simulink model "Regelungsmodell_Roboterarm"  (R2018b)
settings: Solver=VariableStepAuto  StartTime=0.0  StopTime=2  RelTol=1e-3
values from neighbouring files (symbols this model uses):
  konvert_i_torque = 0.11    [Aufgabe_3_Regler.m]
libraries: simulink x2, cstblocks x2
settings Model: Creator=jens  LastModifiedBy=jens

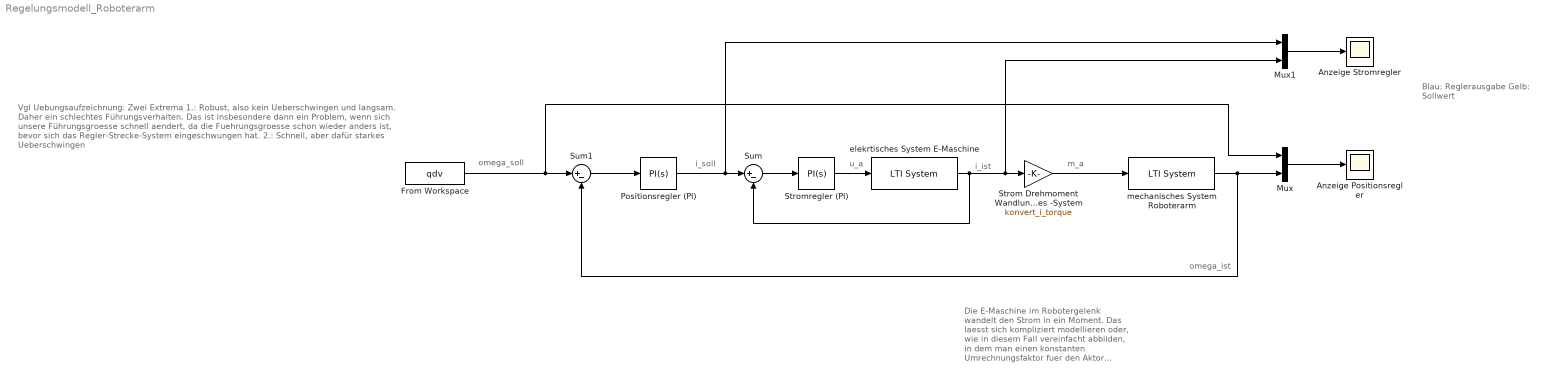
== system Regelungsmodell_Roboterarm ==
  note: Vgl Uebungsaufzeichnung:
      |
      | Zwei Extrema
      |
      | 1.: Robust, also kein Ueberschwingen und langsam. Daher ein schlechtes Führungsverhalten. Das ist insbesondere dann ein Problem, wenn sich unsere Führungsgroesse schnell aendert, da die Fuehrungsgroesse schon wieder anders ist, bevor sich das Regler-Strecke-System eingeschwungen hat.
      |
      | 2.: Schnell, aber dafür starkes Ueberschwingen
  note: m_a
  note: i_ist
  note: u_a
  note: i_soll
  note: omega_soll
  note: omega_ist
  note: Blau:
      | Reglerausgabe
      |
      | Gelb:
      | Sollwert
  note: Die E-Maschine im Robotergelenk wandelt den Strom in ein Moment. Das laesst sich kompliziert modellieren oder, wie in diesem Fall vereinfacht abbilden, in dem man einen konstanten Umrechnungsfaktor fuer den Aktor verwendet.
      | Das ist quasi die Schnittstelle zwischen dem elektrischen Modell und dem mechanischen Modell! Das gestellte Moment m_a ist ueber den Faktor 'konvert_i_torque' direkt proportional zum durch den Stromregler umgesetzten Strom
  Anzeige Positionsregler : Scope
  Anzeige Stromregler : Scope
  From Workspace : FromWorkspace  VariableName=qdv  SampleTime=0
  Mux : Mux  Inputs=2
  Mux1 : Mux  Inputs=2
  Positionsregler (PI) : simulink/Continuous/PID Controller  Controller=PI  Form=Parallel  TimeDomain=Continuous-time  SampleTime=-1  IntegratorMethod=Forward Euler  FilterMethod=Forward Euler  ControllerParametersSource=internal  P=0.150480850040603  I=3  D=0  UseFilter=on  N=100  TunerSelectOption=Transfer Function Based (PID Tuner App)  InitialConditionSource=internal  InitialConditionForIntegrator=0  InitialConditionForFilter=0  DifferentiatorICPrevScaledInput=0  ExternalReset=none  TrackingMode=off  Kt=1  LimitOutput=off  UpperSaturationLimit=inf  LowerSaturationLimit=-inf  LinearizeAsGain=on  AntiWindupMode=none  Kb=1  POutMin=[]  POutMax=[]  IOutMin=[]  IOutMax=[]  DOutMin=[]  DOutMax=[]  NOutMin=[]  NOutMax=[]  SumOutMin=[]  SumOutMax=[]  SaturationOutMin=[]  SaturationOutMax=[]  PParamMin=[]  PParamMax=[]  IParamMin=[]  IParamMax=[]  DParamMin=[]  DParamMax=[]  NParamMin=[]  NParamMax=[]  KbParamMin=[]  KbParamMax=[]  KtParamMin=[]  KtParamMax=[]  KbOutMin=[]  KbOutMax=[]  KtOutMin=[]  KtOutMax=[]  IntegratorOutMin=[]  IntegratorOutMax=[]  FilterOutMin=[]  FilterOutMax=[]  SumI1OutMin=[]  SumI1OutMax=[]  SumI2OutMin=[]  SumI2OutMax=[]  SumI3OutMin=[]  SumI3OutMax=[]  SumI4OutMin=[]  SumI4OutMax=[]  SumDOutMin=[]  SumDOutMax=[]  DifferentiatorOutMin=[]  DifferentiatorOutMax=[]  FilterDiffOutCoefMin=[]  FilterDiffOutCoefMax=[]  ReciprocalOutMin=[]  ReciprocalOutMax=[]  SumDenOutMin=[]  SumDenOutMax=[]  SumNumOutMin=[]  SumNumOutMax=[]  DivideOutMin=[]  DivideOutMax=[]  IntegratorContinuousStateAttributes=''  IntegratorStateMustResolveToSignalObject=off  IntegratorRTWStateStorageClass=Auto  FilterContinuousStateAttributes=''  FilterStateMustResolveToSignalObject=off  FilterRTWStateStorageClass=Auto  ParallelPVariant=InternalParameters  IdealPVariant=Disabled  IVariant=InternalParameters  DVariant=Disabled  IntegratorVariant=Continuous  SatVariant=Disabled  AWVariant=Passthrough  PCopyVariant=Disabled  TRVariant=Disabled  FdbkBlocksVariant=Forward  IdealPFdbkVariant=Disabled  SatFdbkVariant=Disabled  DerivativeFilterVariant=Disabled  NVariant=Disabled  NCopyVariant=Disabled_SignalSpec  FilterICVariant=Disabled  IntegratorICVariant=InternalICs  ExternalResetVariant=Disabled  TRSumVariant=Passthrough  SumFdbkVariant=Disabled  SumVariant=Sum_PI
  "Strom Drehmoment Wandlung - Schnittstelle elektrisches- und mechanisches -System " : Gain  Gain=konvert_i_torque
  Stromregler (PI) : simulink/Continuous/PID Controller  Controller=PI  Form=Parallel  TimeDomain=Continuous-time  SampleTime=-1  IntegratorMethod=Forward Euler  FilterMethod=Forward Euler  ControllerParametersSource=internal  P=0.3  I=3.5  D=0  UseFilter=on  N=100  TunerSelectOption=Transfer Function Based (PID Tuner App)  InitialConditionSource=internal  InitialConditionForIntegrator=0  InitialConditionForFilter=0  DifferentiatorICPrevScaledInput=0  ExternalReset=none  TrackingMode=off  Kt=1  LimitOutput=off  UpperSaturationLimit=inf  LowerSaturationLimit=-inf  LinearizeAsGain=on  AntiWindupMode=none  Kb=1  POutMin=[]  POutMax=[]  IOutMin=[]  IOutMax=[]  DOutMin=[]  DOutMax=[]  NOutMin=[]  NOutMax=[]  SumOutMin=[]  SumOutMax=[]  SaturationOutMin=[]  SaturationOutMax=[]  PParamMin=[]  PParamMax=[]  IParamMin=[]  IParamMax=[]  DParamMin=[]  DParamMax=[]  NParamMin=[]  NParamMax=[]  KbParamMin=[]  KbParamMax=[]  KtParamMin=[]  KtParamMax=[]  KbOutMin=[]  KbOutMax=[]  KtOutMin=[]  KtOutMax=[]  IntegratorOutMin=[]  IntegratorOutMax=[]  FilterOutMin=[]  FilterOutMax=[]  SumI1OutMin=[]  SumI1OutMax=[]  SumI2OutMin=[]  SumI2OutMax=[]  SumI3OutMin=[]  SumI3OutMax=[]  SumI4OutMin=[]  SumI4OutMax=[]  SumDOutMin=[]  SumDOutMax=[]  DifferentiatorOutMin=[]  DifferentiatorOutMax=[]  FilterDiffOutCoefMin=[]  FilterDiffOutCoefMax=[]  ReciprocalOutMin=[]  ReciprocalOutMax=[]  SumDenOutMin=[]  SumDenOutMax=[]  SumNumOutMin=[]  SumNumOutMax=[]  DivideOutMin=[]  DivideOutMax=[]  IntegratorContinuousStateAttributes=''  IntegratorStateMustResolveToSignalObject=off  IntegratorRTWStateStorageClass=Auto  FilterContinuousStateAttributes=''  FilterStateMustResolveToSignalObject=off  FilterRTWStateStorageClass=Auto  ParallelPVariant=InternalParameters  IdealPVariant=Disabled  IVariant=InternalParameters  DVariant=Disabled  IntegratorVariant=Continuous  SatVariant=Disabled  AWVariant=Passthrough  PCopyVariant=Disabled  TRVariant=Disabled  FdbkBlocksVariant=Forward  IdealPFdbkVariant=Disabled  SatFdbkVariant=Disabled  DerivativeFilterVariant=Disabled  NVariant=Disabled  NCopyVariant=Disabled_SignalSpec  FilterICVariant=Disabled  IntegratorICVariant=InternalICs  ExternalResetVariant=Disabled  TRSumVariant=Passthrough  SumFdbkVariant=Disabled  SumVariant=Sum_PI
  Sum : Sum  Inputs=|+-
  Sum1 : Sum  Inputs=|+-
  elekrtisches System E-Maschine : cstblocks/LTI System  sys=tf_motor  IC=[]
  mechanisches System Roboterarm : cstblocks/LTI System  sys=tf_arm  IC=[]
  wires:
  Sum/1 -> Stromregler (PI)/1
  Stromregler (PI)/1 -> elekrtisches System E-Maschine/1
  Positionsregler (PI)/1 -> Mux1/1, Sum/1
  From Workspace/1 -> Mux/1, Sum1/1
  Sum1/1 -> Positionsregler (PI)/1
  mechanisches System Roboterarm/1 -> Sum1/2, Mux/2
  Mux/1 -> Anzeige Positionsregler/1
  "Strom Drehmoment Wandlung - Schnittstelle elektrisches- und mechanisches -System "/1 -> mechanisches System Roboterarm/1
  Mux1/1 -> Anzeige Stromregler/1
  elekrtisches System E-Maschine/1 -> Mux1/2, "Strom Drehmoment Wandlung - Schnittstelle elektrisches- und mechanisches -System "/1, Sum/2
